simulink model "med_sim_ob"  (R2017b)
settings: Solver=ode4  StartTime=0.0  StopTime=100  FixedStep=0.1  RelTol=1e-3
values from neighbouring files (symbols this model uses):
  A = [A11 A12 A13 A14; A21 A22 A23 A24; A31 A32 A33 A34; A41 A42 A43 A44]    [oneforall.m]
  B = [0;0;0;1/jm]    [oneforall.m]
  C = eye(4)    [oneforall.m]
  Kob = place(A,B,Pob)    [oneforall.m]
  L = place(A.',C.',Pob).'    [oneforall.m]
settings Model: Creator=lencs  LastModifiedBy=lencs

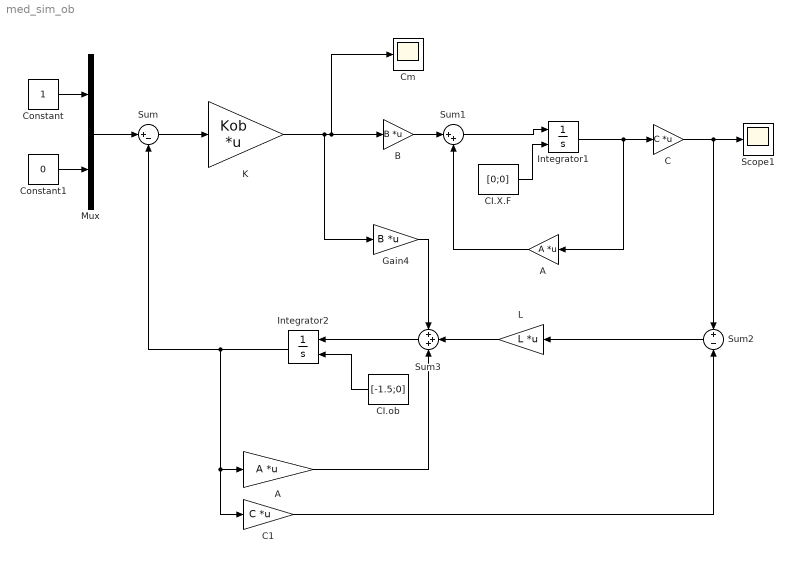
== system med_sim_ob ==
  A : Gain  Gain=A  Multiplication=Matrix(K*u) (u vector)
  "A " : Gain  Gain=A  Multiplication=Matrix(K*u)
  B : Gain  Gain=B  Multiplication=Matrix(K*u)
  C : Gain  Gain=C  Multiplication=Matrix(K*u)
  C1 : Gain  Gain=C  Multiplication=Matrix(K*u)
  CI.X.F : Constant  Value=[0;0]
  CI.ob : Constant  Value=[-1.5;0]
  Cm : Scope
  Constant : Constant
  Constant1 : Constant  Value=0
  Gain4 : Gain  Gain=B  Multiplication=Matrix(K*u)
  Integrator1 : Integrator  InitialConditionSource=external  InitialCondition=[0.1;0;0;0]
  Integrator2 : Integrator  InitialConditionSource=external  InitialCondition=[0.05 ;0; 0; 0]
  K : Gain  Gain=Kob  Multiplication=Matrix(K*u)
  L : Gain  Gain=L  Multiplication=Matrix(K*u)
  Mux : Mux  Inputs=2
  Scope1 : Scope
  Sum : Sum  Inputs=|+-
  Sum1 : Sum  Inputs=|++
  Sum2 : Sum  Inputs=+-
  Sum3 : Sum  Inputs=+++
  wires:
  Constant/1 -> Mux/1
  Mux/1 -> Sum/1
  Sum/1 -> K/1
  Sum1/1 -> Integrator1/1
  Integrator1/1 -> C/1, "A "/1
  C/1 -> Sum2/1, Scope1/1
  "A "/1 -> Sum1/2
  B/1 -> Sum1/1
  Constant1/1 -> Mux/2
  CI.X.F/1 -> Integrator1/2
  K/1 -> Gain4/1, Cm/1, B/1
  A/1 -> Sum3/3
  L/1 -> Sum3/2
  Sum2/1 -> L/1
  Gain4/1 -> Sum3/1
  C1/1 -> Sum2/2
  Integrator2/1 -> A/1, C1/1, Sum/2
  Sum3/1 -> Integrator2/1
  CI.ob/1 -> Integrator2/2
